simulink model "Relay"  (R2022b)
settings: Solver=VariableStepAuto  StartTime=0.0  StopTime=10.0  RelTol=1e-3
undefined symbols (not defined in the file or in its folder): J, k_f, k_v, ke, km, L, R
settings Model: Creator=User  LastModifiedBy=User
settings SolverCC: ZeroCrossAlgorithm=Adaptive
settings DebuggingCC: IgnoredZcDiagnostic=none

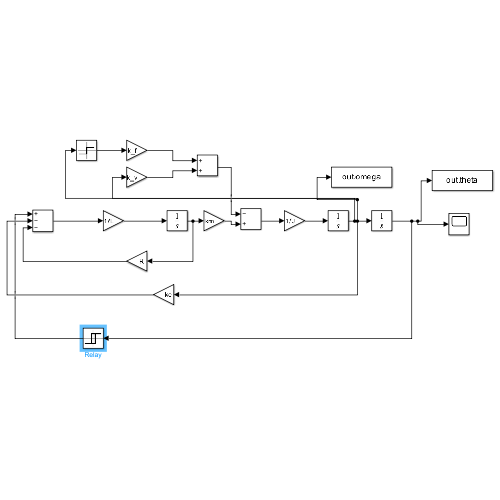
[thumbnail: Simulink's stored preview of the top-level diagram]
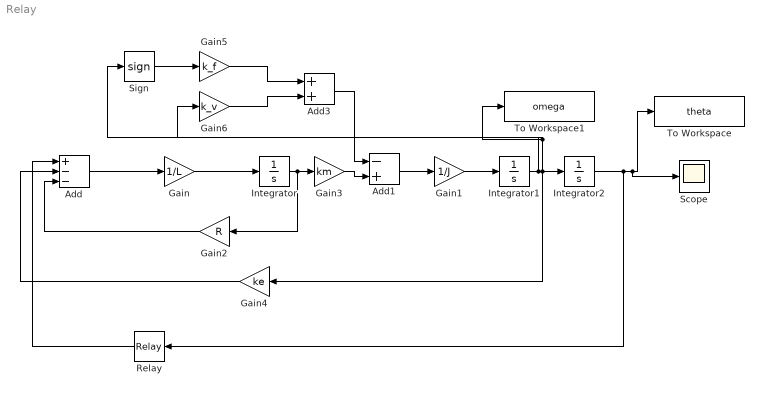
== system Relay ==
  Add : Sum  Inputs=+--
  Add1 : Sum  Inputs=-+
  Add3 : Sum
  Gain : Gain  Gain=1/L
  Gain1 : Gain  Gain=1/J
  Gain2 : Gain  Gain=R
  Gain3 : Gain  Gain=km
  Gain4 : Gain  Gain=ke
  Gain5 : Gain  Gain=k_f
  Gain6 : Gain  Gain=k_v
  Integrator : Integrator
  Integrator1 : Integrator
  Integrator2 : Integrator
  Relay : Relay  OnSwitchValue=0  OffSwitchValue=0  OnOutputValue=-10  OffOutputValue=10
  Scope : Scope
  Sign : Signum
  To Workspace : ToWorkspace  VariableName=theta  SampleTime=-1
  To Workspace1 : ToWorkspace  VariableName=omega  SaveFormat=Timeseries  SampleTime=-1
  wires:
  Add/1 -> Gain/1
  Gain/1 -> Integrator/1
  Integrator/1 -> Gain2/1, Gain3/1
  Add3/1 -> Add1/1
  Gain3/1 -> Add1/2
  Add1/1 -> Gain1/1
  Gain1/1 -> Integrator1/1
  Integrator1/1 -> Gain6/1, Sign/1, To Workspace1/1, Gain4/1, Integrator2/1
  Integrator2/1 -> Relay/1, Scope/1, To Workspace/1
  Gain2/1 -> Add/3
  Gain4/1 -> Add/2
  Sign/1 -> Gain5/1
  Gain6/1 -> Add3/2
  Gain5/1 -> Add3/1
  Relay/1 -> Add/1
